simulink model "depth_multiview_image_200917_r4"  (R2021a)
settings: Solver=FixedStepDiscrete  StartTime=0.0  StopTime=inf  FixedStep=4  RelTol=1e-3  EnableMultiTasking=on
model workspace (MAT data in the model file):
  SL_ROS_VariableLengthArrays_MaxSizes.CommonInfo.ArrayTruncateAction = 'EmitWarning'
  SL_ROS_VariableLengthArrays_MaxSizes.MsgTypeMap = containers.Map
  SL_ROS_VariableLengthArrays_MaxSizes.MsgTypeMap.serialization.keys = {'sensor_msgs/Image', 'sensor_msgs/LaserScan', 'sensor_msgs/PointCloud2', 'std_msgs/Float64MultiArray'}
  SL_ROS_VariableLengthArrays_MaxSizes.MsgTypeMap.serialization.values{1}(1).PropertyName = 'Data'
  SL_ROS_VariableLengthArrays_MaxSizes.MsgTypeMap.serialization.values{1}(1).DataType = 'uint8'
  SL_ROS_VariableLengthArrays_MaxSizes.MsgTypeMap.serialization.values{1}(1).MaxLength = 750000
  SL_ROS_VariableLengthArrays_MaxSizes.MsgTypeMap.serialization.values{1}(2).PropertyName = 'Encoding'
  SL_ROS_VariableLengthArrays_MaxSizes.MsgTypeMap.serialization.values{1}(2).DataType = 'uint8'
  SL_ROS_VariableLengthArrays_MaxSizes.MsgTypeMap.serialization.values{1}(2).MaxLength = 128
  SL_ROS_VariableLengthArrays_MaxSizes.MsgTypeMap.serialization.values{2}(1).PropertyName = 'Intensities'
  SL_ROS_VariableLengthArrays_MaxSizes.MsgTypeMap.serialization.values{2}(1).DataType = 'single'
  SL_ROS_VariableLengthArrays_MaxSizes.MsgTypeMap.serialization.values{2}(1).MaxLength = 360
  SL_ROS_VariableLengthArrays_MaxSizes.MsgTypeMap.serialization.values{2}(2).PropertyName = 'Ranges'
  SL_ROS_VariableLengthArrays_MaxSizes.MsgTypeMap.serialization.values{2}(2).DataType = 'single'
  SL_ROS_VariableLengthArrays_MaxSizes.MsgTypeMap.serialization.values{2}(2).MaxLength = 360
  SL_ROS_VariableLengthArrays_MaxSizes.MsgTypeMap.serialization.values{3}(1).PropertyName = 'Data'
  SL_ROS_VariableLengthArrays_MaxSizes.MsgTypeMap.serialization.values{3}(1).DataType = 'uint8'
  SL_ROS_VariableLengthArrays_MaxSizes.MsgTypeMap.serialization.values{3}(1).MaxLength = 1000000
  SL_ROS_VariableLengthArrays_MaxSizes.MsgTypeMap.serialization.values{3}(2).PropertyName = 'Fields'
  SL_ROS_VariableLengthArrays_MaxSizes.MsgTypeMap.serialization.values{3}(2).DataType = 'sensor_msgs/PointField'
  SL_ROS_VariableLengthArrays_MaxSizes.MsgTypeMap.serialization.values{3}(2).MaxLength = 16
  SL_ROS_VariableLengthArrays_MaxSizes.MsgTypeMap.serialization.values{4}.PropertyName = 'Data'
  SL_ROS_VariableLengthArrays_MaxSizes.MsgTypeMap.serialization.values{4}.DataType = 'double'
  SL_ROS_VariableLengthArrays_MaxSizes.MsgTypeMap.serialization.values{4}.MaxLength = 360
  SL_ROS_VariableLengthArrays_MaxSizes.MsgTypeMap.serialization.uniformity = 0
  SL_ROS_VariableLengthArrays_MaxSizes.MsgTypeMap.serialization.keyType = 'char'
  SL_ROS_VariableLengthArrays_MaxSizes.MsgTypeMap.serialization.valueType = 'any'
undefined symbols (not defined in the file): Data, Data_SL_Info, Encoding, Encoding_SL_Info, Height, IsBigendian, Step, Width
libraries: robotlib x11
settings Model: Creator=USER  LastModifiedBy=note
settings SolverCC: AlgebraicLoopSolver=TrustRegion
settings DataIOCC: ReturnWorkspaceOutputs=off
settings OptimizationCC: StrengthReduction=on  PassReuseOutputArgsAs=Individual arguments  MaxStackSize=64  OptimizeBlockOrder=speed  OptimizationPriority=Speed  OptimizationCustomize=off  MultiThreadedLoops=on  EfficientTunableParamExpr=on
settings DebuggingCC: ParameterTunabilityLossMsg=error  SFMachineParentedDataDiag=warning  ArithmeticOperatorsInVariantConditions=warning
settings HardwareCC: ProdBitPerLong=64  ProdHWDeviceType=Intel->x86-64 (Linux 64)
settings SFSimCC: SimUseLocalCustomCode=off  MATLABDynamicMemAlloc=off  CustomCodeUndefinedFunction=UseInterfaceOnly  SimTargetLang=C++
settings RTWCC: SystemTargetFile=ert.tlc  HardwareBoard=Robot Operating System (ROS)  TLCOptions="-aInlineSetEventsForThisBaseRateFcn=TLC_FALSE -aSuppressMultiTaskScheduler=TLC_FALSE  -aRateBasedStepFcn=0"  TemplateMakefile=ert_default_tmf  GenerateReport=on  RTWUseLocalCustomCode=off  Toolchain=Catkin  BuildConfiguration=Faster Runs  IncludeHyperlinkInReport=on  LaunchReport=on  TargetLang=C++  GenerateTraceInfo=on  GenerateTraceReport=on  GenerateTraceReportSl=on  GenerateTraceReportSf=on  GenerateTraceReportEml=on
settings CodeAppCC: ForceParamTrailComments=on  IgnoreCustomStorageClasses=off  OperatorAnnotations=on  SimulinkDataObjDesc=on  SFDataObjDesc=on  InsertBlockDesc=on
settings ERTTargetCC: SupportVariableSizeSignals=on

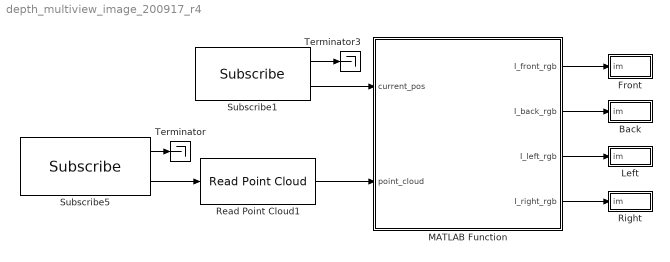
== system depth_multiview_image_200917_r4 ==
  Back : Subsystem
  Front : Subsystem
  Left : Subsystem
  MATLAB Function : MATLAB Function  TreatAsAtomicUnit=on
  Read Point Cloud1 : robotlib/Read Point Cloud  MaximumPointCloudSize=[1, 1000000]  PreserveStructure=off  ShowRGBOutput=off  ShowIntensityOutput=off  ShowErrorCodeOutput=off  VariableSizeOutputs=on
      settings: SourceProductBaseCode=RR
  Right : Subsystem
  Subscribe1 : robotlib/Subscribe  topicSource=Select from ROS network  topic=/rtabmap/odom  messageType=nav_msgs/Odometry  SampleTime=-1  legacyBusStruct=off  messageQueueLength=1
  Subscribe5 : robotlib/Subscribe  topicSource=Select from ROS network  topic=/rtabmap/cloud_map  messageType=sensor_msgs/PointCloud2  SampleTime=-1  legacyBusStruct=off  messageQueueLength=1
  Terminator : Terminator
  Terminator3 : Terminator
  wires:
  Subscribe1/1 -> Terminator3/1
  Subscribe5/2 -> Read Point Cloud1/1
  Subscribe5/1 -> Terminator/1
  ? -> ?
  Subscribe1/2 -> MATLAB Function/1(current_pos)
  Read Point Cloud1/1 -> MATLAB Function/2(point_cloud)
  MATLAB Function/1(I_front_rgb) -> Front/1(im)
  MATLAB Function/2(I_back_rgb) -> Back/1(im)
  MATLAB Function/3(I_left_rgb) -> Left/1(im)
  MATLAB Function/4(I_right_rgb) -> Right/1(im)

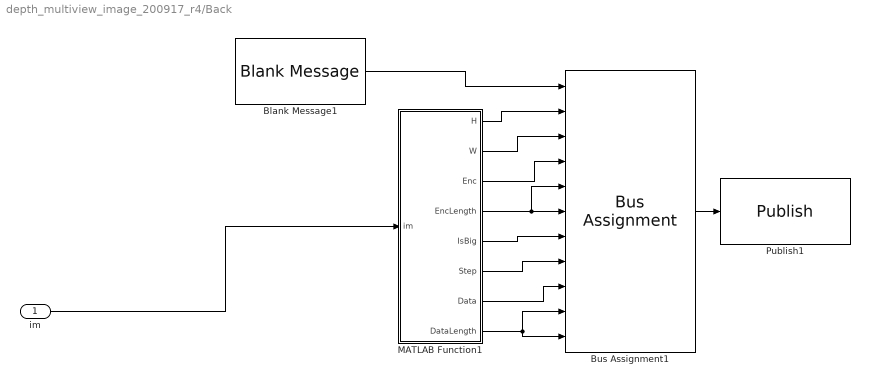
== system depth_multiview_image_200917_r4/Back ==
  im : Inport
  Blank Message1 : robotlib/Blank Message  messageClass=Message  entityType=sensor_msgs/Image  messageType=sensor_msgs/Image  SampleTime=inf  legacyBusStruct=off
  Bus Assignment1 : BusAssignment  AssignedSignals=Height,Width,Encoding,Encoding_SL_Info.CurrentLength,Encoding_SL_Info.ReceivedLength,IsBigendian,Step,Data,Data_SL_Info.CurrentLength,Data_SL_Info.ReceivedLength
  MATLAB Function1 : MATLAB Function  TreatAsAtomicUnit=on
  Publish1 : robotlib/Publish  topicSource=Specify your own  topic=/image_back  messageType=sensor_msgs/Image  legacyBusStruct=off  messageQueueLength=1
  wires:
  Bus Assignment1/1 -> Publish1/1
  MATLAB Function1/6(Step) -> Bus Assignment1/8
  MATLAB Function1/7(Data) -> Bus Assignment1/9
  MATLAB Function1/2(W) -> Bus Assignment1/3
  MATLAB Function1/5(IsBig) -> Bus Assignment1/7
  MATLAB Function1/1(H) -> Bus Assignment1/2
  im/1 -> MATLAB Function1/1(im)
  MATLAB Function1/3(Enc) -> Bus Assignment1/4
  MATLAB Function1/8(DataLength) -> Bus Assignment1/10, Bus Assignment1/11
  Blank Message1/1 -> Bus Assignment1/1
  MATLAB Function1/4(EncLength) -> Bus Assignment1/6, Bus Assignment1/5

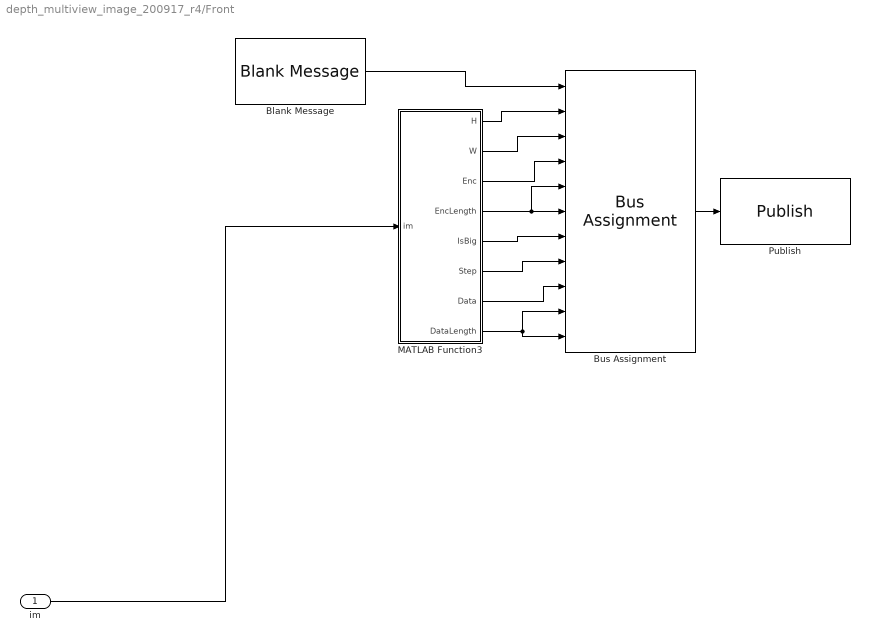
== system depth_multiview_image_200917_r4/Front ==
  im : Inport
  Blank Message : robotlib/Blank Message  messageClass=Message  entityType=sensor_msgs/Image  messageType=sensor_msgs/Image  SampleTime=inf  legacyBusStruct=off
  Bus Assignment : BusAssignment  AssignedSignals=Height,Width,Encoding,Encoding_SL_Info.CurrentLength,Encoding_SL_Info.ReceivedLength,IsBigendian,Step,Data,Data_SL_Info.CurrentLength,Data_SL_Info.ReceivedLength
  MATLAB Function3 : MATLAB Function  TreatAsAtomicUnit=on
  Publish : robotlib/Publish  topicSource=Specify your own  topic=/image_front  messageType=sensor_msgs/Image  legacyBusStruct=off  messageQueueLength=1
  wires:
  Bus Assignment/1 -> Publish/1
  MATLAB Function3/3(Enc) -> Bus Assignment/4
  Blank Message/1 -> Bus Assignment/1
  MATLAB Function3/5(IsBig) -> Bus Assignment/7
  im/1 -> MATLAB Function3/1(im)
  MATLAB Function3/8(DataLength) -> Bus Assignment/10, Bus Assignment/11
  MATLAB Function3/7(Data) -> Bus Assignment/9
  MATLAB Function3/2(W) -> Bus Assignment/3
  MATLAB Function3/1(H) -> Bus Assignment/2
  MATLAB Function3/4(EncLength) -> Bus Assignment/6, Bus Assignment/5
  MATLAB Function3/6(Step) -> Bus Assignment/8

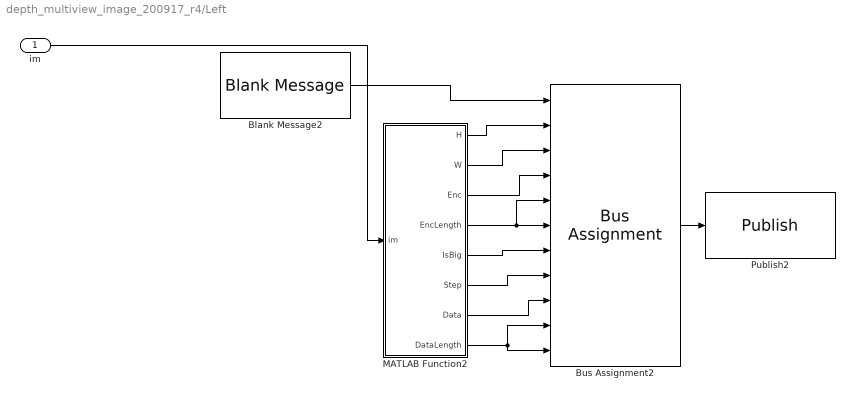
== system depth_multiview_image_200917_r4/Left ==
  im : Inport
  Blank Message2 : robotlib/Blank Message  messageClass=Message  entityType=sensor_msgs/Image  messageType=sensor_msgs/Image  SampleTime=inf  legacyBusStruct=off
  Bus Assignment2 : BusAssignment  AssignedSignals=Height,Width,Encoding,Encoding_SL_Info.CurrentLength,Encoding_SL_Info.ReceivedLength,IsBigendian,Step,Data,Data_SL_Info.CurrentLength,Data_SL_Info.ReceivedLength
  MATLAB Function2 : MATLAB Function  TreatAsAtomicUnit=on
  Publish2 : robotlib/Publish  topicSource=Specify your own  topic=/image_left  messageType=sensor_msgs/Image  legacyBusStruct=off  messageQueueLength=1
  wires:
  Blank Message2/1 -> Bus Assignment2/1
  Bus Assignment2/1 -> Publish2/1
  MATLAB Function2/1(H) -> Bus Assignment2/2
  MATLAB Function2/4(EncLength) -> Bus Assignment2/6, Bus Assignment2/5
  MATLAB Function2/5(IsBig) -> Bus Assignment2/7
  MATLAB Function2/3(Enc) -> Bus Assignment2/4
  MATLAB Function2/2(W) -> Bus Assignment2/3
  im/1 -> MATLAB Function2/1(im)
  MATLAB Function2/6(Step) -> Bus Assignment2/8
  MATLAB Function2/8(DataLength) -> Bus Assignment2/10, Bus Assignment2/11
  MATLAB Function2/7(Data) -> Bus Assignment2/9

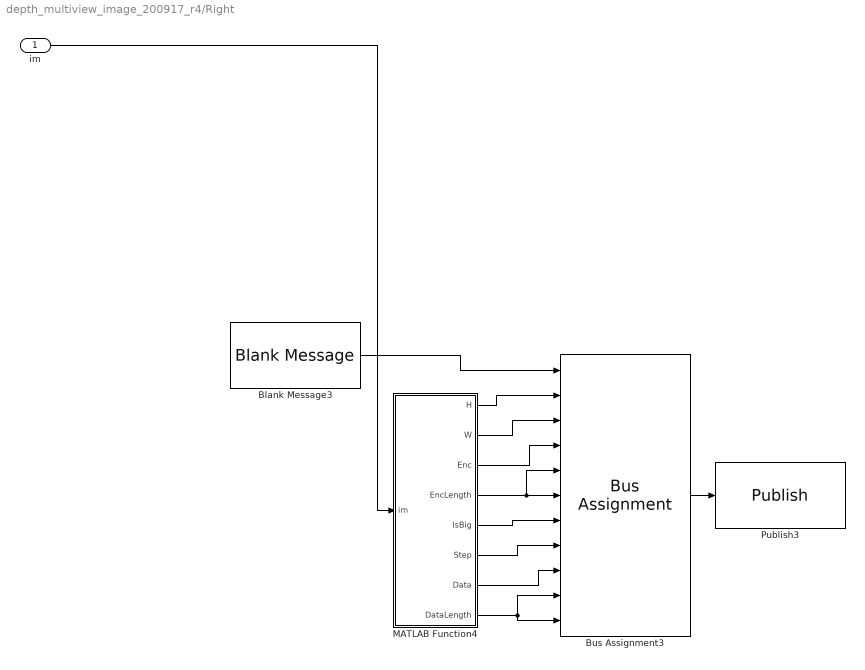
== system depth_multiview_image_200917_r4/Right ==
  im : Inport
  Blank Message3 : robotlib/Blank Message  messageClass=Message  entityType=sensor_msgs/Image  messageType=sensor_msgs/Image  SampleTime=inf  legacyBusStruct=off
  Bus Assignment3 : BusAssignment  AssignedSignals=Height,Width,Encoding,Encoding_SL_Info.CurrentLength,Encoding_SL_Info.ReceivedLength,IsBigendian,Step,Data,Data_SL_Info.CurrentLength,Data_SL_Info.ReceivedLength
  MATLAB Function4 : MATLAB Function  TreatAsAtomicUnit=on
  Publish3 : robotlib/Publish  topicSource=Specify your own  topic=/image_right  messageType=sensor_msgs/Image  legacyBusStruct=off  messageQueueLength=1
  wires:
  MATLAB Function4/5(IsBig) -> Bus Assignment3/7
  MATLAB Function4/1(H) -> Bus Assignment3/2
  MATLAB Function4/6(Step) -> Bus Assignment3/8
  MATLAB Function4/2(W) -> Bus Assignment3/3
  MATLAB Function4/8(DataLength) -> Bus Assignment3/10, Bus Assignment3/11
  Blank Message3/1 -> Bus Assignment3/1
  MATLAB Function4/3(Enc) -> Bus Assignment3/4
  MATLAB Function4/7(Data) -> Bus Assignment3/9
  im/1 -> MATLAB Function4/1(im)
  MATLAB Function4/4(EncLength) -> Bus Assignment3/6, Bus Assignment3/5
  Bus Assignment3/1 -> Publish3/1

== matlab function depth_multiview_image_200917_r4/Back/MATLAB Function1 ==
  data: H output; im input; W output; Enc output; EncLength output; IsBig output; Step output; Data output; DataLength output
function [H, W, Enc, EncLength, IsBig, Step, Data, DataLength] = fcn(im)
  [H, W, n] = size(im);
  H =uint32(H); W =uint32(W);
  im = permute(im,[2 1 3]);
  Data1 = im(:);
  Data2 = reshape(Data1,[H*W,n])';
  Data = Data2(:);
  Data = uint8(Data*255);
  Enc = zeros(1,128, 'uint8');
  Enc(1:4) = uint8('rgb8'); %   uint8('rgb8')
  EncLength = uint32(4);
  IsBig = uint8(0);
  Step = uint32(W*n);
  DataLength = uint32(H*W*n);


% % % % function [Height,Width,Encoding,Image]   = func(data)
% % % % % test = single(nan(1,128));
% % % % Height = 500;
% % % % Width = 500;
% % % % Image = single(data);
% % % % % for i = 1:length(data)
% % % % %     test(i) = single(data(i));
% % % % % end
% % % % Encoding = 'rgb8';
% % % % SL = uint32(numel(data));
% % % % 
% % % % 
% % % % end

== matlab function depth_multiview_image_200917_r4/MATLAB Function ==
  data: current_pos input; I_front_rgb output; point_cloud input; I_back_rgb output; I_left_rgb output; I_right_rgb output
function [I_front_rgb,I_back_rgb,I_left_rgb,I_right_rgb] = fcn(current_pos,point_cloud)
% function I_front_rgb  = fcn(current_pos,point_cloud)

% persistent image_hz image_temp_front image_temp_back image_temp_left image_temp_right
%     pos_x = current_pos.Poses(end).Pose.Position.X;
%     pos_y = current_pos.Poses(end).Pose.Position.Y;
%     pos_z = current_pos.Poses(end).Pose.Position.Z;
    
pos_x = current_pos.Pose.Pose.Position.X;
pos_y = current_pos.Pose.Pose.Position.Y;
pos_z = current_pos.Pose.Pose.Position.Z;

image_grid = 0.02;                           %m
image_size = 500;
distance=4;

for lll=1:numel(point_cloud)/3
    if sqrt((point_cloud(lll,1)-pos_x)^2 + (point_cloud(lll,2)-pos_y)^2 + (point_cloud(lll,3)-pos_z)^2) > distance
        point_cloud(lll,:)=nan(1,3);
    else
        point_cloud(lll,:)=[point_cloud(lll,1)-pos_x, point_cloud(lll,2)-pos_y, point_cloud(lll,3)-pos_z];
    end
end

% point = rmmissing(point_cloud);
point = point_cloud;


% if isempty(image_hz)
%     image_hz = 299;
% end
% if isempty(image_temp_front)
%     image_temp_front = single(cat(3,zeros(image_size,image_size),zeros(image_size,image_size),zeros(image_size,image_size)));
% end
% if isempty(image_temp_back)
%     image_temp_back = single(cat(3,zeros(image_size,image_size),zeros(image_size,image_size),zeros(image_size,image_size)));
% end
% if isempty(image_temp_left)
%     image_temp_left = single(cat(3,zeros(image_size,image_size),zeros(image_size,image_size),zeros(image_size,image_size)));
% end
% if isempty(image_temp_right)
%     image_temp_right = single(cat(3,zeros(image_size,image_size),zeros(image_size,image_size),zeros(image_size,image_size)));
% end
% 
% image_hz = image_hz + 1;
% 
% % tic
% if image_hz == 300
%     image_hz = 1;


% indices_front = cell(image_size,image_size);
% indices_back = cell(image_size,image_size);
% indices_right = cell(image_size,image_size);
% indices_left = cell(image_size,image_size);
indices_front = zeros(image_size,image_size);
indices_back = zeros(image_size,image_size);
indices_right = zeros(image_size,image_size);
indices_left = zeros(image_size,image_size);

% if ~(current_pos(1) == 0 && current_pos(2) == 0 && current_pos(3) == 0)
    
    size = numel(point)/3;
    point_shifted = point+image_size*image_grid/2;
    % point_grided = int16(point.Location/test_grid);
    point_grided = int16(point_shifted/image_grid);
%     
%     current_x = pos_x/test_grid;
%     current_y = pos_y/test_grid;
%     current_z = pos_z/test_grid;
%     
%     for aa = 1:size
%         if point(aa,1) >= pos_x
%             indices_front{point_grided(aa,3),point_grided(aa,2)}=[indices_front{point_grided(aa,3),point_grided(aa,2)};aa];
%         elseif point(aa,1) <= pos_x
%             indices_back{point_grided(aa,3),point_grided(aa,2)}=[indices_back{point_grided(aa,3),point_grided(aa,2)};aa];
%         end
%         
%         if point(aa,2) >= pos_y
%             indices_left{point_grided(aa,3),point_grided(aa,1)}=[indices_left{point_grided(aa,3),point_grided(aa,1)};aa];
%         elseif point(aa,2) <= pos_y
%             indices_right{point_grided(aa,3),point_grided(aa,1)}=[indices_right{point_grided(aa,3),point_grided(aa,1)};aa];
%         end
%     end
    
    for aa = 1:size
%         if point(aa,1) >= pos_x
        if point(aa,1) >= 0
            indices_front(point_grided(aa,3),point_grided(aa,2))=1;
%         elseif point(aa,1) <= pos_x
        elseif point(aa,1) <= 0
            indices_back(point_grided(aa,3),point_grided(aa,2))=1;
        end
        
%         if point(aa,2) >= pos_y
        if point(aa,2) >= 0
            indices_left(point_grided(aa,3),point_grided(aa,1))=1;
%         elseif point(aa,2) <= pos_y
        elseif point(aa,2) <= 0
            indices_right(point_grided(aa,3),point_grided(aa,1))=1;
        end
    end
    
    I_front = flip(flip(indices_front,1),2);
    I_back = flip(flip(indices_back,1),2);
    I_left = flip(indices_left,1);
    I_right = flip(indices_right,1);
    
%     I_front_rgb = single(cat(3,cat(3,I_front,I_front),I_front));
%     I_back_rgb = single(cat(3,cat(3,I_back,I_back),I_back));
%     I_left_rgb = single(cat(3,cat(3,I_left,I_left),I_left));
%     I_right_rgb = single(cat(3,cat(3,I_right,I_right),I_right));
    
    image_temp_front = single(cat(3,cat(3,I_front,I_front),I_front));
    image_temp_back = single(cat(3,cat(3,I_back,I_back),I_back));
    image_temp_left = single(cat(3,cat(3,I_left,I_left),I_left));
    image_temp_right = single(cat(3,cat(3,I_right,I_right),I_right));
    
% end

    I_front_rgb = image_temp_front;
    I_back_rgb = image_temp_back;
    I_left_rgb = image_temp_left;
    I_right_rgb = image_temp_right;
%     point_filtered=point_cloud;

== matlab function depth_multiview_image_200917_r4/Front/MATLAB Function3 ==
  data: H output; im input; W output; Enc output; EncLength output; IsBig output; Step output; Data output; DataLength output
function [H, W, Enc, EncLength, IsBig, Step, Data, DataLength] = fcn(im)
  [H, W, n] = size(im);
  H =uint32(H); W =uint32(W);
  im = permute(im,[2 1 3]);
  Data1 = im(:);
  Data2 = reshape(Data1,[H*W,n])';
  Data = Data2(:);
  Data = uint8(Data*255);
  Enc = zeros(1,128, 'uint8');
  Enc(1:4) = uint8('rgb8'); %   uint8('rgb8')
  EncLength = uint32(4);
  IsBig = uint8(0);
  Step = uint32(W*n);
  DataLength = uint32(H*W*n);


% % % % function [Height,Width,Encoding,Image]   = func(data)
% % % % % test = single(nan(1,128));
% % % % Height = 500;
% % % % Width = 500;
% % % % Image = single(data);
% % % % % for i = 1:length(data)
% % % % %     test(i) = single(data(i));
% % % % % end
% % % % Encoding = 'rgb8';
% % % % SL = uint32(numel(data));
% % % % 
% % % % 
% % % % end

== matlab function depth_multiview_image_200917_r4/Left/MATLAB Function2 ==
  data: H output; im input; W output; Enc output; EncLength output; IsBig output; Step output; Data output; DataLength output
function [H, W, Enc, EncLength, IsBig, Step, Data, DataLength] = fcn(im)
  [H, W, n] = size(im);
  H =uint32(H); W =uint32(W);
  im = permute(im,[2 1 3]);
  Data1 = im(:);
  Data2 = reshape(Data1,[H*W,n])';
  Data = Data2(:);
  Data = uint8(Data*255);
  Enc = zeros(1,128, 'uint8');
  Enc(1:4) = uint8('rgb8'); %   uint8('rgb8')
  EncLength = uint32(4);
  IsBig = uint8(0);
  Step = uint32(W*n);
  DataLength = uint32(H*W*n);


% % % % function [Height,Width,Encoding,Image]   = func(data)
% % % % % test = single(nan(1,128));
% % % % Height = 500;
% % % % Width = 500;
% % % % Image = single(data);
% % % % % for i = 1:length(data)
% % % % %     test(i) = single(data(i));
% % % % % end
% % % % Encoding = 'rgb8';
% % % % SL = uint32(numel(data));
% % % % 
% % % % 
% % % % end

== matlab function depth_multiview_image_200917_r4/Right/MATLAB Function4 ==
  data: H output; im input; W output; Enc output; EncLength output; IsBig output; Step output; Data output; DataLength output
function [H, W, Enc, EncLength, IsBig, Step, Data, DataLength] = fcn(im)
  [H, W, n] = size(im);
  H =uint32(H); W =uint32(W);
  im = permute(im,[2 1 3]);
  Data1 = im(:);
  Data2 = reshape(Data1,[H*W,n])';
  Data = Data2(:);
  Data = uint8(Data*255);
  Enc = zeros(1,128, 'uint8');
  Enc(1:4) = uint8('rgb8'); %   uint8('rgb8')
  EncLength = uint32(4);
  IsBig = uint8(0);
  Step = uint32(W*n);
  DataLength = uint32(H*W*n);


% % % % function [Height,Width,Encoding,Image]   = func(data)
% % % % % test = single(nan(1,128));
% % % % Height = 500;
% % % % Width = 500;
% % % % Image = single(data);
% % % % % for i = 1:length(data)
% % % % %     test(i) = single(data(i));
% % % % % end
% % % % Encoding = 'rgb8';
% % % % SL = uint32(numel(data));
% % % % 
% % % % 
% % % % end
